simulink subsystem "drivetrain"  (R2021a)
settings: Solver=VariableStepAuto  StartTime=0.0  StopTime=10.0  RelTol=1e-3
values from neighbouring files (symbols this model uses):
  InverterParRes = 10000    [drivetrain_ws.m]
  InverterRes = 0    [drivetrain_ws.m]
libraries: fl_lib x6, nesl_utility x3
settings Model: Creator=Carlo Edoardo  LastModifiedBy=miche

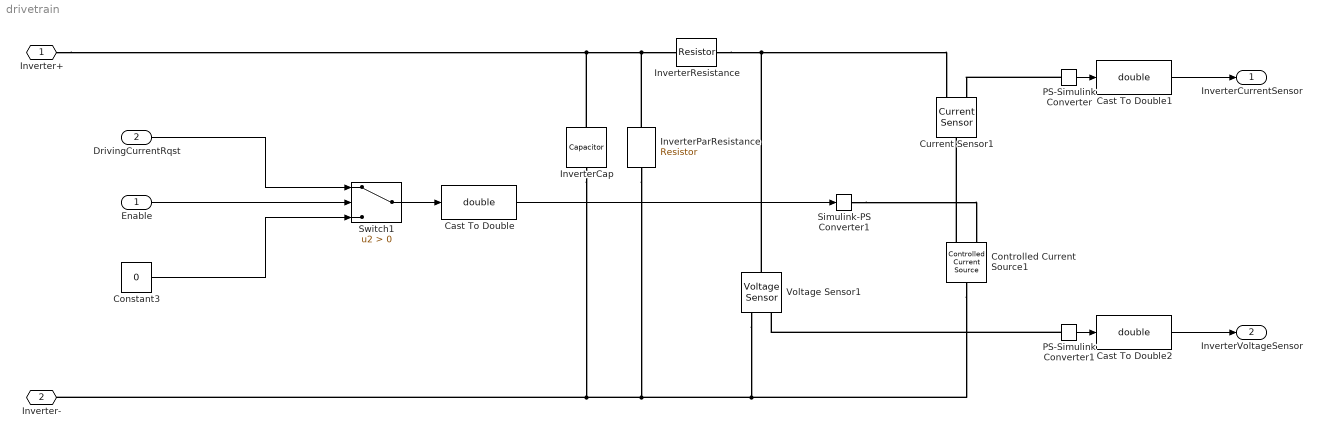
== system drivetrain ==
  Enable : Inport
  DrivingCurrentRqst : Inport  Port=2
  Cast To Double : DataTypeConversion  OutDataTypeStr=double
  Cast To Double1 : DataTypeConversion  OutDataTypeStr=double
  Cast To Double2 : DataTypeConversion  OutDataTypeStr=double
  Constant3 : Constant  Value=0
  Controlled Current Source1 : fl_lib/Electrical/Electrical Sources/Controlled Current Source
  Current Sensor1 : fl_lib/Electrical/Electrical Sensors/Current Sensor
  InverterCap : fl_lib/Electrical/Electrical Elements/Capacitor  c=InverterCap F  r=1e-6 Ohm  g=0 1/Ohm  i_specify=off  i_priority=None  i=0 A  i_nominal_specify=off  i_nominal_unit=A  i_nominal_value=1  v_specify=off  v_priority=None  v=0 V  v_nominal_specify=off  v_nominal_unit=V  v_nominal_value=1  vc_specify=off  vc_priority=High  vc=0 V  vc_nominal_specify=off  vc_nominal_unit=V  vc_nominal_value=1
  InverterParResistance : fl_lib/Electrical/Electrical Elements/Resistor  R=InverterParRes Ohm  i_specify=off  i_priority=None  i=0 A  i_nominal_specify=off  i_nominal_unit=A  i_nominal_value=1  v_specify=off  v_priority=None  v=0 V  v_nominal_specify=off  v_nominal_unit=V  v_nominal_value=1
  InverterResistance : fl_lib/Electrical/Electrical Elements/Resistor  R=InverterRes Ohm  i_specify=off  i_priority=None  i=0 A  i_nominal_specify=off  i_nominal_unit=A  i_nominal_value=1  v_specify=off  v_priority=None  v=0 V  v_nominal_specify=off  v_nominal_unit=V  v_nominal_value=1
  PS-Simulink Converter : nesl_utility/PS-Simulink Converter  PhysicalDomain=network_engine_domain  SubClassName=ps_output  LeftPortType=input  RightPortType=output  PseudoPeriodic=off  Frequencies=[]  Unit=inherit  AffineConversion=off
      settings: SourceProductBaseCode=PW,SS
  PS-Simulink Converter1 : nesl_utility/PS-Simulink Converter  PhysicalDomain=network_engine_domain  SubClassName=ps_output  LeftPortType=input  RightPortType=output  PseudoPeriodic=off  Frequencies=[]  Unit=inherit  AffineConversion=off
      settings: SourceProductBaseCode=PW,SS
  Simulink-PS Converter1 : nesl_utility/Simulink-PS Converter  PhysicalDomain=network_engine_domain  SubClassName=ps_input  LeftPortType=input  RightPortType=output  PseudoPeriodic=off  Frequencies=[]  NoiseDistribution=none  NoiseParameters=[]  Unit=1  AffineConversion=off  FilteringAndDerivatives=provide  SimscapeFilterOrder=1  InputFilterTimeConstant=0.001  UdotUserProvided=0
      settings: SourceProductBaseCode=PW,SS
  Switch1 : Switch  Criteria=u2 > Threshold
  Voltage Sensor1 : fl_lib/Electrical/Electrical Sensors/Voltage Sensor
  Inverter+ : PMIOPort  Side=Left
  Inverter- : PMIOPort  Port=2  Side=Left
  InverterCurrentSensor : Outport
  InverterVoltageSensor : Outport  Port=2
  wires:
  Switch1/1 -> Cast To Double/1
  Constant3/1 -> Switch1/3
  DrivingCurrentRqst/1 -> Switch1/1
  Cast To Double/1 -> Simulink-PS Converter1/1
  PS-Simulink Converter1/1 -> Cast To Double2/1
  Cast To Double2/1 -> InverterVoltageSensor/1
  PS-Simulink Converter/1 -> Cast To Double1/1
  Cast To Double1/1 -> InverterCurrentSensor/1
  Enable/1 -> Switch1/2
  connections:
  Voltage Sensor1/RConn2 -- Controlled Current Source1/LConn1 -- Inverter-/RConn1 -- InverterCap/RConn1 -- InverterParResistance/RConn1
  InverterResistance/RConn1 -- Current Sensor1/RConn2 -- Voltage Sensor1/LConn1
  InverterCap/LConn1 -- Inverter+/RConn1 -- InverterResistance/LConn1 -- InverterParResistance/LConn1
  Simulink-PS Converter1/RConn1 -- Controlled Current Source1/RConn1
  Controlled Current Source1/RConn2 -- Current Sensor1/LConn1
  PS-Simulink Converter1/LConn1 -- Voltage Sensor1/RConn1
  PS-Simulink Converter/LConn1 -- Current Sensor1/RConn1
